simulink model "Observador"  (R2021a)
settings: Solver=ode45  StartTime=0.0  StopTime=10  RelTol=1e-3  EnableMultiTasking=on
values from neighbouring files (symbols this model uses):
  A = [0 1 0;0 0 1;-6 -11 -6]    [Projeto_observador.m]    (also in Q1_OBS.m = [0 1; -50 -15]; Q2_OBS.m = [0 0 -150; 1 0 -95;  0 1 -18]; exemplo.m = [0 1 0; 0 0 1; -6 -11 -6])
  B = [0 0 1]'    [Projeto_observador.m]    (also in Q1_OBS.m = [0 1]'; Q2_OBS.m = [150; 1; 0]; exemplo.m = [0; 0; 1])
  C = [1 0 0]    [Projeto_observador.m]    (also in Q1_OBS.m = [2 1]; Q2_OBS.m = [0 0 1]; exemplo.m)
  Ke = acker(A',C',autovaloresOBSV)'    [Projeto_observador.m]    (also in Q1_OBS.m = acker(A', C', autovaloresOBSV)'; Q2_OBS.m = acker(A', C', autovaloresOBSV)'; exemplo.m = acker(A', C', autovaloresOBSV)')
settings Model: Creator=Rafael Cardoso  LastModifiedBy=wesll
settings SolverCC: AlgebraicLoopSolver=TrustRegion
settings DataIOCC: LimitDataPoints=on  SaveFormat=Array  SignalLoggingSaveFormat=ModelDataLogs  ReturnWorkspaceOutputs=off
settings OptimizationCC: ExpressionDepthLimit=2147483647  LifeSpan=inf
settings DebuggingCC: UnderspecifiedInitializationDetection=Classic  MergeDetectMultiDrivingBlocksExec=none  SolverPrmCheckMsg=warning  FcnCallInpInsideContextMsg=warning  StateNameClashWarn=warning  SFUnexpectedBacktrackingDiag=warning  SFNoUnconditionalDefaultTransitionDiag=warning  SFExecutionAtInitializationDiag=none  SFMachineParentedDataDiag=warning  ArithmeticOperatorsInVariantConditions=warning
settings HardwareCC: ProdBitPerPointer=32  ProdBitPerSizeT=32  ProdBitPerPtrDiffT=32  ProdLargestAtomicFloat=None  ProdIntDivRoundTo=Undefined  ProdEndianess=Unspecified  ProdWordSize=32  ProdHWDeviceType=32-bit Generic
settings ModelReferenceCC: PropagateSignalLabelsOutOfModel=off
settings SFSimCC: SimUseLocalCustomCode=off  CustomCodeUndefinedFunction=UseInterfaceOnly
settings RTWCC: RTWUseLocalCustomCode=off
settings CodeAppCC: StateflowObjectComments=on
settings GRTTargetCC: TargetLangStandard=C89/C90 (ANSI)  CombineOutputUpdateFcns=off  GRTInterface=on
settings ConfigComp: CovMetricSettings=dw  CovSaveCumulativeToWorkspaceVar=on  CovSaveSingleToWorkspaceVar=on  CovExternalEMLEnable=off

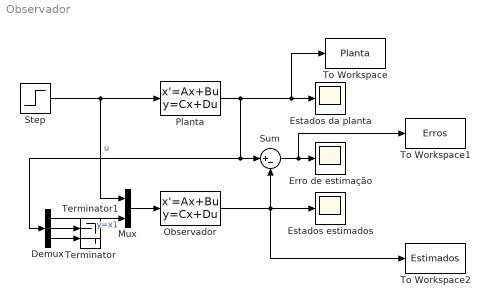
== system Observador ==
  Demux : Demux  Outputs=3
  Erro de estimação : Scope
  Estados da planta : Scope
  Estados estimados : Scope
  Mux : Mux  Inputs=2
  Observador : StateSpace  A=(A-Ke*C)  B=[B Ke]  C=eye(3)  D=zeros(3,2)  InitialCondition=[0 0 0]
  Planta : StateSpace  A=A  B=B  C=eye(3)  D=zeros(3,1)  InitialCondition=[1 -1 0.5]
  Step : Step  Time=0  After=10  SampleTime=0
  Sum : Sum  Inputs=|+-
  Terminator : Terminator
  Terminator1 : Terminator
  To Workspace : ToWorkspace  VariableName=Planta  SaveFormat=Structure With Time  SampleTime=-1
  To Workspace1 : ToWorkspace  VariableName=Erros  SaveFormat=Structure With Time  SampleTime=-1
  To Workspace2 : ToWorkspace  VariableName=Estimados  SaveFormat=Structure With Time  SampleTime=-1
  wires:
  Step/1 -> Planta/1, Mux/1  "u"
  Mux/1 -> Observador/1
  Observador/1 -> To Workspace2/1, Estados estimados/1, Sum/2
  Planta/1 -> To Workspace/1, Estados da planta/1, Demux/1, Sum/1
  Sum/1 -> To Workspace1/1, Erro de estimação/1
  Demux/1 -> Mux/2  "y=x1"
  Demux/2 -> Terminator1/1
  Demux/3 -> Terminator/1
